simulink model "TestSim"  (R2016a)
settings: Solver=VariableStepAuto  StartTime=0.0  StopTime=inf  RelTol=1e-3
StartFcn:
  | %EventListener
  | h = add_exec_event_listener('TestSim/Product','PostOutputs',@EventListener);
libraries: sldrtlib x1, aerolibanimutils x1
settings Model: Creator=zhan.xiong  LastModifiedBy=ccc

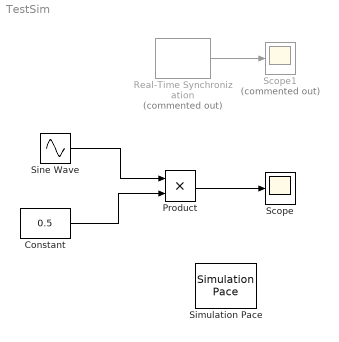
== system TestSim ==
  Constant : Constant  Value=0.5
  Product : Product
  Real-Time Synchronization : sldrtlib/Real-Time Synchronization  Commented=on  SampleTime=0.1  MaxMissedTicks=inf  ShowMissedTicks=on  YieldWhenWaiting=on
  Scope : Scope
  Scope1 : Scope  Commented=on
  Simulation Pace : aerolibanimutils/Simulation Pace  SimulationPace=1  SleepMode=MATLAB Thread  OutputPaceError=off  SampleTime=1/30
  Sine Wave : Sin  SampleTime=0
  wires:
  Product/1 -> Scope/1
  Sine Wave/1 -> Product/1
  Constant/1 -> Product/2
  Real-Time Synchronization/1 -> Scope1/1
